simulink model "PardoSplitTwo"  (R2023b)
settings: Solver=VariableStepAuto  StartTime=0.0  StopTime=10.0  RelTol=1e-3
settings Model: Creator=jsonm  LastModifiedBy=jsonm

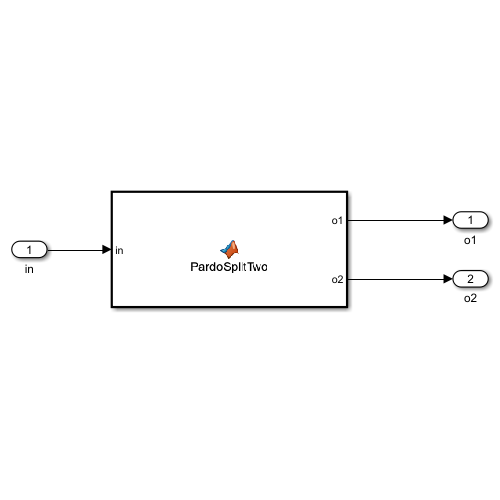
[thumbnail: Simulink's stored preview of the top-level diagram]
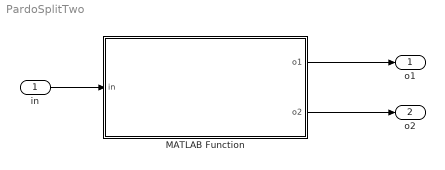
== system PardoSplitTwo ==
  in : Inport
  MATLAB Function : MATLAB Function  TreatAsAtomicUnit=on
  o1 : Outport
  o2 : Outport  Port=2
  wires:
  in/1 -> MATLAB Function/1(in)
  MATLAB Function/1(o1) -> o1/1
  MATLAB Function/2(o2) -> o2/1

== matlab function PardoSplitTwo/MATLAB Function ==
  data: in input; o1 output; o2 output
function [o1, o2] = PardoSplitTwo(in)

% Method to demux input into one of two possible outputs based on assumption
% that processes run in parallel and they must all complete.
%
% Non-valid output is negative
%
% Written by: Darian Muresan
% Modified by: Jason McCauley

if in < 0
        o1 = -1;
        o2 = -1;
else
        o1 = in;
        o2 = in;
end
